simulink model "model"  (R2024a)
settings: Solver=FixedStepAuto  StartTime=0.0  StopTime=10.0  FixedStep=0.001  RelTol=1e-3
settings Model: Creator=main  LastModifiedBy=main

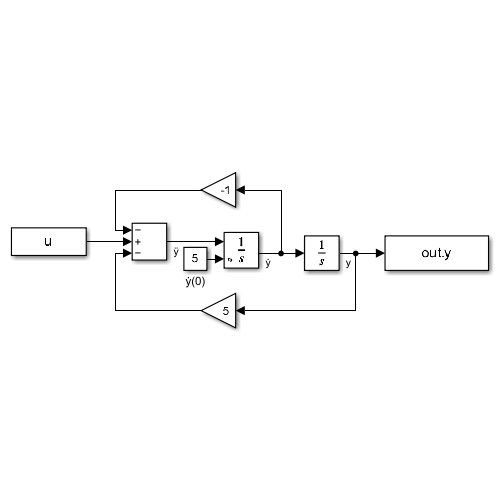
[thumbnail: Simulink's stored preview of the top-level diagram]
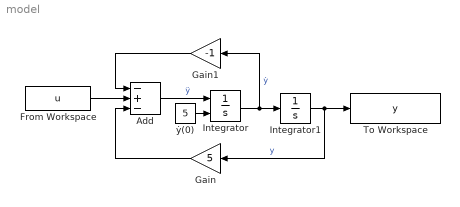
== system model ==
  Add : Sum  Inputs=-+-
  From Workspace : FromWorkspace  VariableName=u
  Gain : Gain  Gain=5
  Gain1 : Gain  Gain=-1
  Integrator : Integrator  InitialConditionSource=external  InitialCondition=5
  Integrator1 : Integrator
  To Workspace : ToWorkspace  VariableName=y  SaveFormat=Timeseries  SampleTime=-1
  ẏ(0) : Constant  Value=5
  wires:
  From Workspace/1 -> Add/2
  Add/1 -> Integrator/1  "ÿ"
  Integrator/1 -> Gain1/1, Integrator1/1  "ẏ"
  Integrator1/1 -> To Workspace/1, Gain/1  "y"
  Gain/1 -> Add/3
  Gain1/1 -> Add/1
  ẏ(0)/1 -> Integrator/2
